simulink model "Feedforward"  (R2022b)
settings: Solver=FixedStepAuto  StartTime=0.0  StopTime=10.0  MaxStep=0.1  RelTol=1e-3
undefined symbols (not defined in the file): unicycle
libraries: simulink_extras x1
settings Model: Creator=hp 2021  LastModifiedBy=Musta
settings ModelReferenceCC: EnableRefExpFcnMdlSchedulingChecks=on

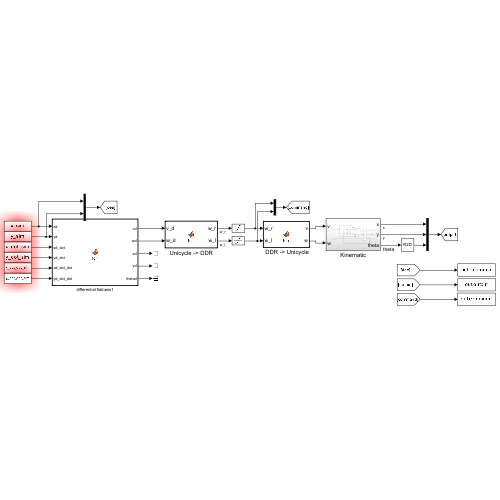
[thumbnail: Simulink's stored preview of the top-level diagram]
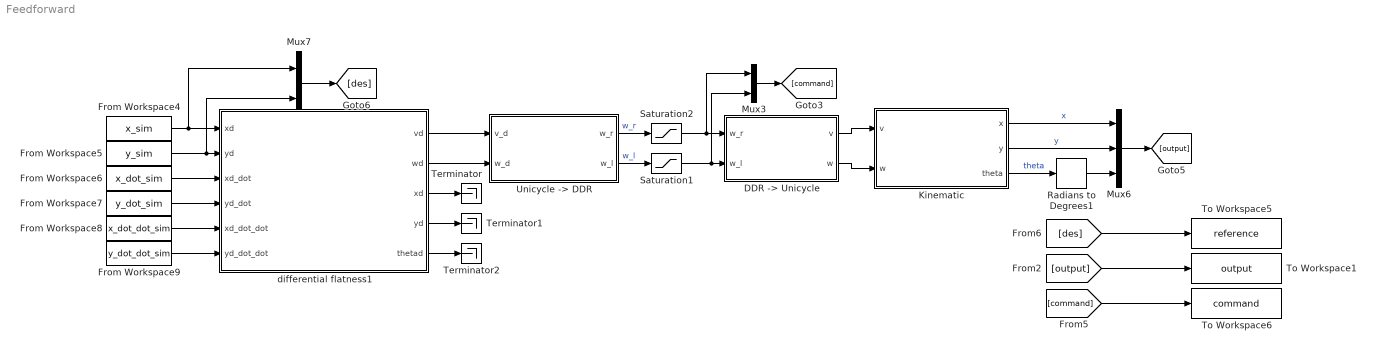
== system Feedforward ==
  " DDR -> Unicycle" : MATLAB Function  TreatAsAtomicUnit=on
  From Workspace4 : FromWorkspace  VariableName=x_sim
  From Workspace5 : FromWorkspace  VariableName=y_sim
  From Workspace6 : FromWorkspace  VariableName=x_dot_sim
  From Workspace7 : FromWorkspace  VariableName=y_dot_sim
  From Workspace8 : FromWorkspace  VariableName=x_dot_dot_sim
  From Workspace9 : FromWorkspace  VariableName=y_dot_dot_sim
  Kinematic : Subsystem
  Mux3 : Mux  Inputs=2
  Mux6 : Mux  Inputs=3
  Mux7 : Mux  Inputs=2
  Radians to Degrees1 : simulink_extras/Transformations/Radians to Degrees
  Saturation1 : Saturate  UpperLimit=unicycle.omegaWheelMax  LowerLimit=unicycle.omegaWheelMin
  Saturation2 : Saturate  UpperLimit=unicycle.omegaWheelMax  LowerLimit=unicycle.omegaWheelMin
  Terminator : Terminator
  Terminator1 : Terminator
  Terminator2 : Terminator
  To Workspace1 : ToWorkspace  VariableName=output  SaveFormat=Structure With Time  SampleTime=-1
  To Workspace5 : ToWorkspace  VariableName=reference  SaveFormat=Structure With Time  SampleTime=-1
  To Workspace6 : ToWorkspace  VariableName=command  SaveFormat=Structure With Time  SampleTime=-1
  "Unicycle -> DDR" : MATLAB Function  TreatAsAtomicUnit=on
  differential flatness1 : MATLAB Function  TreatAsAtomicUnit=on
  wires:
  From Workspace8/1 -> differential flatness1/5(xd_dot_dot)
  differential flatness1/2(wd) -> "Unicycle -> DDR"/2(w_d)
  differential flatness1/1(vd) -> "Unicycle -> DDR"/1(v_d)
  differential flatness1/5(thetad) -> Terminator2/1
  From Workspace9/1 -> differential flatness1/6(yd_dot_dot)
  From Workspace7/1 -> differential flatness1/4(yd_dot)
  differential flatness1/4(yd) -> Terminator1/1
  From Workspace6/1 -> differential flatness1/3(xd_dot)
  differential flatness1/3(xd) -> Terminator/1
  Kinematic/2(y) -> Mux6/2  "y"
  Saturation2/1 -> Mux3/1, " DDR -> Unicycle"/1(w_r)
  Mux3/1 -> [command]
  "Unicycle -> DDR"/1(w_r) -> Saturation2/1  "w_r"
  " DDR -> Unicycle"/1(v) -> Kinematic/1(v)
  Kinematic/1(x) -> Mux6/1  "x"
  " DDR -> Unicycle"/2(w) -> Kinematic/2(w)
  "Unicycle -> DDR"/2(w_l) -> Saturation1/1  "w_l"
  Kinematic/3(theta) -> Radians to Degrees1/1  "theta"
  Radians to Degrees1/1 -> Mux6/3
  [output] -> To Workspace1/1
  [command] -> To Workspace6/1
  Saturation1/1 -> Mux3/2, " DDR -> Unicycle"/2(w_l)
  Mux6/1 -> [output]
  From Workspace4/1 -> Mux7/1, differential flatness1/1("xd ")
  Mux7/1 -> [des]
  From Workspace5/1 -> Mux7/2, differential flatness1/2("yd ")
  [des] -> To Workspace5/1

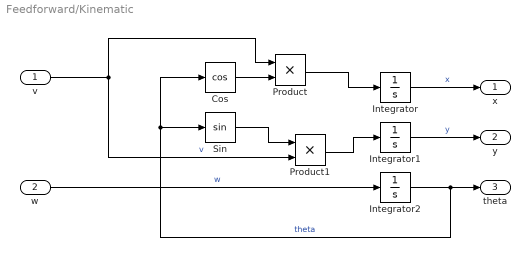
== system Feedforward/Kinematic ==
  v : Inport
  w : Inport  Port=2
  Cos : Trigonometry  Operator=cos
  Integrator : Integrator  InitialCondition=unicycle.ic.x
  Integrator1 : Integrator  InitialCondition=unicycle.ic.y
  Integrator2 : Integrator  InitialCondition=unicycle.ic.theta
  Product : Product
  Product1 : Product
  Sin : Trigonometry
  x : Outport
  y : Outport  Port=2
  theta : Outport  Port=3
  wires:
  w/1 -> Integrator2/1  "w"
  Product/1 -> Integrator/1
  v/1 -> Product/1, Product1/2  "v"
  Cos/1 -> Product/2
  Integrator1/1 -> y/1  "y"
  Integrator/1 -> x/1  "x"
  Integrator2/1 -> Cos/1, Sin/1, theta/1  "theta"
  Product1/1 -> Integrator1/1
  Sin/1 -> Product1/1

== matlab function Feedforward/ DDR -> Unicycle ==
  data: w_r input; v output; w_l input; w output
function [v, w] = fcn(w_r, w_l)

    %#codegen
    coder.extrinsic('evalin')
    d = 0;                  % Needed in order to set variable class correctly
    r = 0;                  % Needed in order to set variable class correctly
    d = evalin('base','unicycle.d'); % Read value from workspace
    r = evalin('base','unicycle.r'); % Read value from workspace

    v = r*(w_r + w_l)/2; % rad/s
    w = r*(w_r - w_l)/d; % rad/s

end

== matlab function Feedforward/Unicycle -> DDR ==
  data: v_d input; w_r output; w_d input; w_l output
function [w_r, w_l] = fcn(v_d, w_d)

    %#codegen
    coder.extrinsic('evalin')
    d = 0;                  % Needed in order to set variable class correctly
    r = 0;                  % Needed in order to set variable class correctly
    d = evalin('base','unicycle.d'); % Read value from workspace
    r = evalin('base','unicycle.r'); % Read value from workspace

    w_r = ((2 * v_d) + (w_d * d)) / (2 * r);
    w_l = ((2 * v_d) - (w_d * d)) / (2 * r);

end

== matlab function Feedforward/differential flatness1 ==
  data: xd input; vd output; yd input; xd_dot input; yd_dot input; xd_dot_dot input; yd_dot_dot input; wd output; xd output; yd output; thetad output
function [vd, wd, xd, yd, thetad] = fcn(xd, yd, xd_dot, yd_dot, xd_dot_dot, yd_dot_dot)
    
    vd = sqrt(xd_dot.^2 + yd_dot.^2);
    wd = (xd_dot.*yd_dot_dot - xd_dot_dot.*yd_dot) / (xd_dot.^2 + yd_dot.^2);
    % thetad = atan2(yd_dot, xd_dot);
    thetad = mod(atan2(yd_dot,xd_dot), 2*pi);

    xd = xd;
    yd = yd;

end
